simulink model "ClosedLoopTest2"  (R2024b)
settings: Solver=FixedStepAuto  StartTime=0.0  StopTime=60  FixedStep=T  MaxStep=0.015  RelTol=1e-3
StopFcn:
  | stopHeli_allTasks
  | daqreset
model workspace: external: MAT-File (data not in the file)
undefined symbols (not defined in the file or in its folder): Discrete, ElevAxisData, K_lqr, PitchAxisData, T, Time
libraries: ctrlSharedLib x1, sldrtlib x1
settings Model: Creator=msciola  LastModifiedBy=leeta
settings SolverCC: AlgebraicLoopSolver=TrustRegion
settings DebuggingCC: UnconnectedInputMsg=warning  UnconnectedOutputMsg=warning  UnconnectedLineMsg=warning
settings ModelReferenceCC: EnableRefExpFcnMdlSchedulingChecks=on
settings SFSimCC: CustomCodeUndefinedFunction=UseInterfaceOnly
settings RTWCC: GPUComputeCapability=3.5

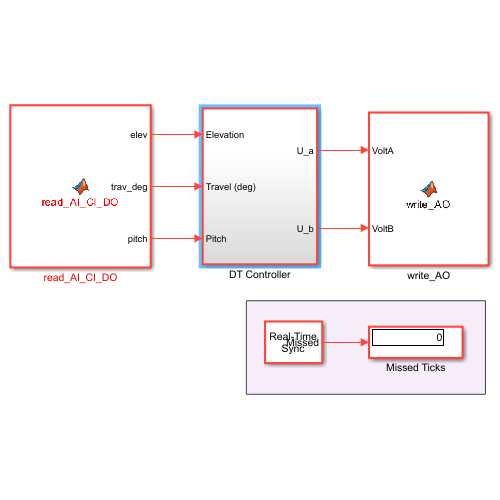
[thumbnail: Simulink's stored preview of the top-level diagram]
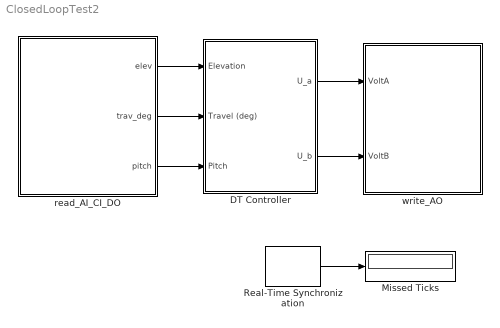
== system ClosedLoopTest2 ==
  DT Controller : Subsystem
  Missed Ticks : Display
  Real-Time Synchronization : sldrtlib/Real-Time Synchronization  SampleTime=T  MaxMissedTicks=inf  ShowMissedTicks=on  YieldWhenWaiting=off
  read_AI_CI_DO : MATLAB Function  TreatAsAtomicUnit=on
  write_AO : MATLAB Function  TreatAsAtomicUnit=on
  wires:
  Real-Time Synchronization/1 -> Missed Ticks/1
  read_AI_CI_DO/3(pitch) -> DT Controller/3(Pitch)
  read_AI_CI_DO/1(elev) -> DT Controller/1(Elevation)
  read_AI_CI_DO/2(trav_deg) -> DT Controller/2(Travel (deg))
  DT Controller/2(U_b) -> write_AO/2(VoltB)
  DT Controller/1(U_a) -> write_AO/1(VoltA)

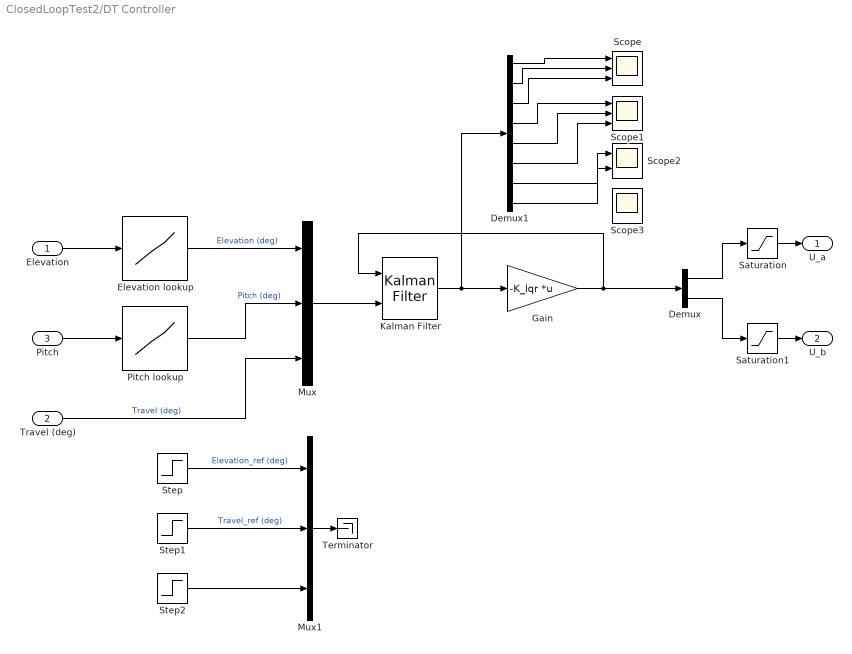
== system ClosedLoopTest2/DT Controller ==
  Elevation : Inport
  Travel (deg) : Inport  Port=2
  Pitch : Inport  Port=3
  " Pitch lookup" : Lookup_n-D  NumberOfTableDimensions=1  LookupTableObject=PitchAxisData  BreakpointsForDimension1=PitchAxisData.Var2  Table=PitchAxisData.Var1  InternalRulePriority=Speed  RndMeth=Simplest
  Demux : Demux  Outputs=2
  Demux1 : Demux  Outputs=nx
  Elevation lookup : Lookup_n-D  NumberOfTableDimensions=1  LookupTableObject=PitchAxisData  BreakpointsForDimension1=ElevAxisData.Var2  Table=ElevAxisData.Var1  InternalRulePriority=Speed  RndMeth=Simplest
  Gain : Gain  Gain=-K_lqr  Multiplication=Matrix(K*u)
  Kalman Filter : ctrlSharedLib/Kalman Filter  TimeDomain=Discrete-Time  UseCurrentEstimator=on  ModelSource=LTI State-Space Variable  ModelSourceVariable=sysdt  A=0.95  B=1  C=1  D=0  NumberOfStates=1  NumberOfInputs=1  NumberOfOutputs=1  InitialEstimateSource=Dialog  X0=0  P0=10  UseK=off  UseGH=off  NumberOfProcessNoiseInputs=1  G=1  TimeInvariantG=on  H=0  TimeInvariantH=on  Q=0.05  TimeInvariantQ=on  R=1  TimeInvariantR=on  N=0  TimeInvariantN=on  AddInputPort=on  AddEnablePort=off  OutputEstimatedY=off  OutputP=off  Ts=-1
  Mux : Mux  Inputs=3
  Mux1 : Mux  Inputs=3
  Saturation : Saturate  UpperLimit=10  LowerLimit=3
  Saturation1 : Saturate  UpperLimit=10  LowerLimit=3
  Scope : Scope  NumInputPorts=3
  Scope1 : Scope  NumInputPorts=3
  Scope2 : Scope  NumInputPorts=2
  Scope3 : Scope  NumInputPorts=2
  Step : Step  Time=0  After=0  SampleTime=T
  Step1 : Step  Time=0  After=0  SampleTime=T
  Step2 : Step  Time=0  After=0  SampleTime=T
  Terminator : Terminator
  U_a : Outport
  U_b : Outport  Port=2
  wires:
  Step2/1 -> Mux1/3
  Elevation/1 -> Elevation lookup/1
  Pitch/1 -> " Pitch lookup"/1
  Elevation lookup/1 -> Mux/1  "Elevation (deg)"
  " Pitch lookup"/1 -> Mux/2  "Pitch (deg)"
  Travel (deg)/1 -> Mux/3  "Travel (deg)"
  Demux/1 -> Saturation/1
  Demux/2 -> Saturation1/1
  Step1/1 -> Mux1/2  "Travel_ref (deg)"
  Step/1 -> Mux1/1  "Elevation_ref (deg)"
  Gain/1 -> Kalman Filter/1, Demux/1
  Mux/1 -> Kalman Filter/2
  Kalman Filter/1 -> Demux1/1, Gain/1
  Mux1/1 -> Terminator/1
  Saturation/1 -> U_a/1
  Saturation1/1 -> U_b/1
  Demux1/1 -> Scope/1
  Demux1/2 -> Scope/2
  Demux1/3 -> Scope/3
  Demux1/4 -> Scope1/1
  Demux1/5 -> Scope1/2
  Demux1/6 -> Scope1/3
  Demux1/7 -> Scope2/1
  Demux1/8 -> Scope2/2

== matlab function ClosedLoopTest2/read_AI_CI_DO ==
  data: elev output; trav_deg output; pitch output
function [elev,trav_deg,pitch] = read_AI_CI_DO()
% The functions from the NI library to read and write inputs and outpus 
% cannot be compiled and we need to use the coder.extrinsic.
% Functions in common to all 
coder.extrinsic('NI_DAQmxCreateTask','NI_DAQmxStartTask','assignin');
%Functions to read AI
coder.extrinsic('daq.ni.NIDAQmx.DAQmx_Val_Diff','NI_DAQmxCreateAIVoltageChan',...
    'NI_DAQmxReadAnalogF64');
%Functions to read CI
coder.extrinsic('NI_DAQmxCreateCILinEncoderChan','NI_DAQmxReadCounterScalarF64',... 
    'daq.ni.NIDAQmx.DAQmx_Val_X1','daq.ni.NIDAQmx.DAQmx_Val_Ticks');
%Functions to write DO
coder.extrinsic('NI_DAQmxWriteDigitalLines','NI_DAQmxCreateDOChan');

%% Configuration
% Specify channels
channelNameAI = {'myDAQ1/ai0','myDAQ1/ai1'};
channelNameCI = 'myDAQ1/ctr0';
channelNamesDO = {'myDAQ1/Port0/Line5', 'myDAQ1/Port0/Line6','myDAQ1/Port0/Line7'};

% Initialize variables for MATLAB Function block to work
elev = 0;
pitch = 0;
numChannels = 1;
trav = zeros(1, numChannels);
y = zeros(1, numChannels);
% make the taskhandle for each channel persistent
persistent taskHandleAI taskHandleCI taskHandleDO
% Create and start tasks for each channel
if isempty(taskHandleAI)
    taskHandleAI = NI_DAQmxCreateTask;
    NI_DAQmxCreateAIVoltageChan(taskHandleAI, channelNameAI{1}, daq.ni.NIDAQmx.DAQmx_Val_Diff, -10, 10)
    NI_DAQmxCreateAIVoltageChan(taskHandleAI, channelNameAI{2}, daq.ni.NIDAQmx.DAQmx_Val_Diff, -10, 10)
    NI_DAQmxStartTask(taskHandleAI);
    assignin('base','taskHandleAI',taskHandleAI);
end
if isempty(taskHandleCI)
    taskHandleCI = NI_DAQmxCreateTask;
    NI_DAQmxCreateCILinEncoderChan( taskHandleCI, channelNameCI, daq.ni.NIDAQmx.DAQmx_Val_X1, daq.ni.NIDAQmx.DAQmx_Val_Ticks, 1); % Check X4 (Labview) or X1 with Bryn
    NI_DAQmxStartTask(taskHandleCI)
    assignin('base','taskHandleCI',taskHandleCI);
end
if isempty (taskHandleDO)
    taskHandleDO = NI_DAQmxCreateTask;
    for ii = 1:numel(channelNamesDO)
        NI_DAQmxCreateDOChan(taskHandleDO, channelNamesDO{ii});
    end
    %numChannelsDO = NI_DAQmxGetWriteNumChans(taskHandleDO);
    NI_DAQmxStartTask(taskHandleDO)
    assignin('base','taskHandleDO',taskHandleDO);
end
%% Read and write channels
% Write the digital outputs
outputData = [0 1 0];
NI_DAQmxWriteDigitalLines(taskHandleDO, outputData);
% Read analog inputs (elevation and pitch angles)
data = NI_DAQmxReadAnalogF64(taskHandleAI,1,2);
elev = data(1);
pitch = data(2);

% Read the counter encoder input (tavel angle)
y = NI_DAQmxReadCounterScalarF64(taskHandleCI);
% To avoid insignificant numbers in the reading
if y> 2^31
    y = y- 2^32;
end
% Transform the encoder reading into angle degrees between 0 and 360
 trav_deg = y*360/500;

== matlab function ClosedLoopTest2/write_AO ==
  data: VoltA input; VoltB input
function write_AO(VoltA,VoltB)
% The functions from the NI library to write outpus cannot be compiled 
% and we need to use the coder.extrinsic.
% Functions in common to all  
coder.extrinsic('NI_DAQmxCreateTask','NI_DAQmxStartTask', 'assignin');
% Functions to write AO
coder.extrinsic('NI_DAQmxCreateAOVoltageChan','NI_DAQmxWriteAnalogF64',...
    'daq.ni.NIDAQmx.DAQmx_Val_Volts');
%% Configuration
% Specify channel
channelNameAO = {'myDAQ1/ao0','myDAQ1/ao1'};
% make the taskhandle persistent
persistent  taskHandleAO 
% Create and start tasks for each channel
if isempty(taskHandleAO)
    taskHandleAO = NI_DAQmxCreateTask;
    NI_DAQmxCreateAOVoltageChan(taskHandleAO, channelNameAO{1})
    NI_DAQmxCreateAOVoltageChan(taskHandleAO, channelNameAO{2})
    NI_DAQmxStartTask(taskHandleAO);
    assignin('base','taskHandleAO',taskHandleAO);
end
%% Write Digital output
NI_DAQmxWriteAnalogF64(taskHandleAO,[VoltA,VoltB]);
end
